simulink model "exp8_1"  (R2023a)
settings: Solver=VariableStepAuto  StartTime=0.0  StopTime=10.0  RelTol=1e-3
libraries: simulink x1
settings Model: Creator=Lenovo  LastModifiedBy=zt

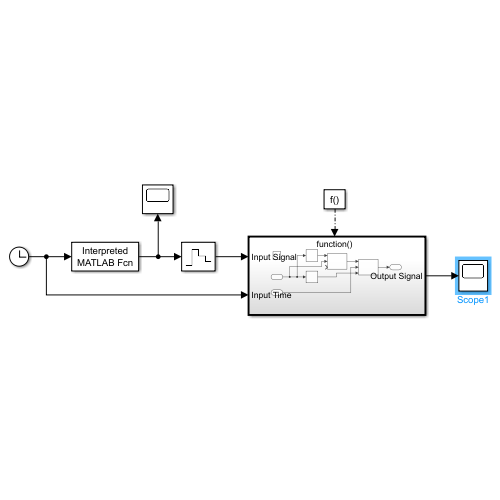
[thumbnail: Simulink's stored preview of the top-level diagram]
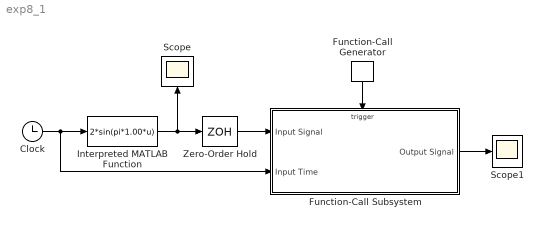
== system exp8_1 ==
  Clock : Clock
  Function-Call Generator : simulink/Ports & Subsystems/Function-Call Generator  sample_time=1/10000  numberOfIterations=1  DisallowWideOutput=off
  Function-Call Subsystem : Subsystem  TreatAsAtomicUnit=on
  Interpreted MATLAB Function : MATLABFcn  MATLABFcn=2*sin(pi*1.00*u)
  Scope : Scope
  Scope1 : Scope
  Zero-Order Hold : ZeroOrderHold  SampleTime=1/10000
  wires:
  Interpreted MATLAB Function/1 -> Zero-Order Hold/1, Scope/1
  Function-Call Subsystem/1(Output Signal) -> Scope1/1
  Function-Call Generator/1 -> Function-Call Subsystem/Trigger
  Zero-Order Hold/1 -> Function-Call Subsystem/1(Input Signal)
  Clock/1 -> Function-Call Subsystem/2(Input Time), Interpreted MATLAB Function/1

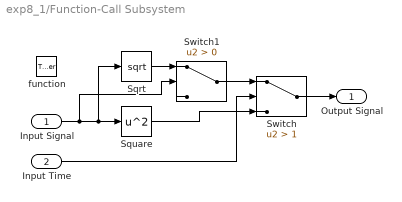
== system exp8_1/Function-Call Subsystem ==
  Input Signal : Inport
  Input Time : Inport  Port=2
  function : TriggerPort  TriggerType=function-call  VariantControl=(inherit)
  Sqrt : Sqrt
  Square : Math  Operator=square
  Switch : Switch  Criteria=u2 > Threshold  Threshold=1  SaturateOnIntegerOverflow=off  InputSameDT=off
  Switch1 : Switch  Criteria=u2 > Threshold  SaturateOnIntegerOverflow=off  InputSameDT=off
  Output Signal : Outport
  wires:
  Input Time/1 -> Switch/2
  Input Signal/1 -> Sqrt/1, Square/1, Switch1/2
  Square/1 -> Switch/3
  Switch/1 -> Output Signal/1
  Sqrt/1 -> Switch1/1
  Switch1/1 -> Switch/1
